simulink model "VehicleFollowing"  (R2020b)
settings: Solver=VariableStepAuto  StartTime=0.0  StopTime=50  RelTol=1e-3
undefined symbols (not defined in the file or in its folder): Discrete, Time
libraries: sim3dautolib x3, vrlib x2, simulink x2, ctrlSharedLib x2, mpcadaslib x2, pid_lib x2, sim3dlib x1, robotmobilelib x1
(part 1 of 2)
settings Model: Creator=Mustafa  LastModifiedBy=JiangHeng
settings SFSimCC: CustomCodeUndefinedFunction=UseInterfaceOnly

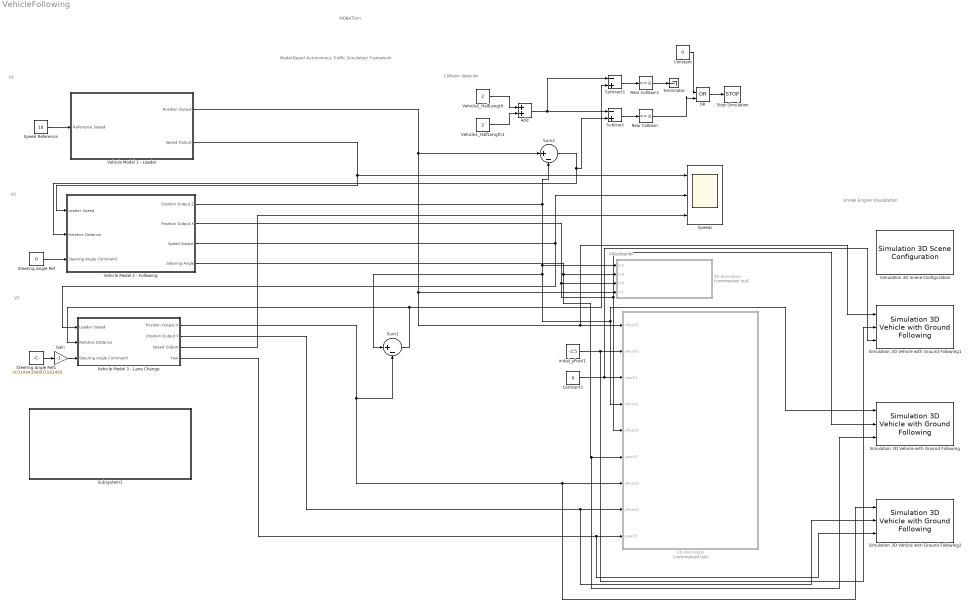
== system VehicleFollowing ==
  note: Unreal Engine Visualization
  note: V1
  note: Visualization
  note: Collision detecion
  note: Model-Based Autonomous Traffic Simulation Framework
  note: MOBATSim
  note: V2
  note: V3
  2D Animation : Subsystem  Commented=on  TreatAsAtomicUnit=on  SystemSampleTime=0.02
  3D Animation : Subsystem  Commented=on
  Add : Sum
  Constant : Constant  Value=0
  Constant1 : Constant  Value=0
  Gain : Gain  Gain=-1
  OR : Logic  Operator=OR  IconShape=distinctive  AllPortsSameDT=off  OutDataTypeStr=boolean
  Rear Collision : simulink/Logic and Bit Operations/Compare To Constant  relop=<=  const=0  OutDataTypeStr=boolean
  Rear Collision1 : simulink/Logic and Bit Operations/Compare To Constant  relop=<=  const=0  OutDataTypeStr=boolean
  Simulation 3D Scene Configuration : sim3dlib/Simulation 3D Scene Configuration  Priority=0  ProjectFormat=Default Scenes  SceneDesc=Straight road  ProjectName=VehicleSimulation.exe  ScenePath=/Game/Maps/HwStrght  vehTagList={'Scene Origin';'SimulinkVehicle1';'SimulinkVehicle2';'SimulinkVehicle3'}  vehTag=SimulinkVehicle3  OpVisEn=off  Ts=0.1  EnableWindow=on  sensorTag=MainCamera1  sensorId=1  sensorName=MainCamera1  mountLoc=Origin  offsetFlag=off  tmountOffset=[0, 0, 0]  rmountOffset=[0, 0, 0]  HorizontalResolution=1280  VerticalResolution=720  HorizontalFOV=60  mountPoint=[0 0 0]  mountOrientation=[0 0 0]  aMode=3  ID=1
      settings: SourceProductBaseCode=DR,UV,VE
  Simulation 3D Vehicle with Ground Following : sim3dautolib/Simulation 3D Vehicle with Ground Following  Priority=-1  PassVehMesh=Small pickup truck  VehColor=Orange  InitialPos=[20, 0, 0]  InitialRot=[0, 0, 0]  ActorName=SimulinkVehicle1  SampleTime=0.1  ActorType=SimulinkVehicle  ID=1  aMode=3  ActorTag=SimulinkVehicle1  CoordinateScheme=ISO  TransformOutportEnabled=off
      settings: SourceProductBaseCode=DR,UV,VE
  Simulation 3D Vehicle with Ground Following1 : sim3dautolib/Simulation 3D Vehicle with Ground Following  Priority=-1  PassVehMesh=Muscle car  VehColor=Red  InitialPos=[40, 0, 0]  InitialRot=[0, 0, 0]  ActorName=SimulinkVehicle2  SampleTime=0.1  ActorType=SimulinkVehicle  ID=2  aMode=3  ActorTag=SimulinkVehicle2  CoordinateScheme=ISO  TransformOutportEnabled=off
      settings: SourceProductBaseCode=DR,UV,VE
  Simulation 3D Vehicle with Ground Following2 : sim3dautolib/Simulation 3D Vehicle with Ground Following  Priority=-1  PassVehMesh=Sedan  VehColor=Silver  InitialPos=[0, 0, 0]  InitialRot=[0, 0, 0]  ActorName=SimulinkVehicle3  SampleTime=0.1  ActorType=SimulinkVehicle  ID=3  aMode=3  ActorTag=SimulinkVehicle3  CoordinateScheme=ISO  TransformOutportEnabled=off
      settings: SourceProductBaseCode=DR,UV,VE
  Speed Reference : Constant  Value=10
  Speeds : Scope  NumInputPorts=3
  Steering Angle Ref : Constant  Value=0
  Steering Angle Ref1 : Constant  Value=-0.01094399007161456
  Stop Simulation : Stop
  Subsystem1 : Subsystem
  Subtract : Sum  Inputs=-+
  Subtract1 : Sum  Inputs=-+
  Sum1 : Sum  Inputs=|+-
  Sum2 : Sum  Inputs=|+-
  Terminator : Terminator
  Vehicle Model 1 - Leader : Subsystem  mask{Pos=40, Speed=20, Disturbance=0}
      mask prompts: Pos "Initial Position"; Speed "Initial Speed"; Disturbance "Leader Vehicle Acceleration Disturbance"
      mask TypeOptions Pos: Initial Position/Value
      mask TypeOptions Speed: Initial Speed/Value
      mask TypeOptions Disturbance: Sine Wave/Amplitude
  Vehicle Model 2 - Following : Subsystem  mask{Pos=20, Speed=25}
      mask prompts: Pos "Initial Position"; Speed "Initial Speed"
      mask TypeOptions Pos: Initial Position Z/Value
      mask TypeOptions Speed: Initial Speed/Value
  Vehicle Model 3 - Lane Change : Subsystem  mask{Pos=0, Speed=10}
      mask prompts: Pos "Initial Position"; Speed "Initial Speed"
      mask TypeOptions Pos: Initial Position X/Value
      mask TypeOptions Speed: Initial Speed/Value
  Vehicle1_HalfLength1 : Constant  Value=2
  Vehicle2_HalfLength : Constant  Value=2
  initial_yPosV1 : Constant  Value=-2.5
  wires:
  Vehicle Model 2 - Following/1(Position Output Z) -> Sum1/1, 2D Animation/4(xPosV2), Simulation 3D Vehicle with Ground Following/1, 3D Animation/1(In2), Sum2/2
  Vehicle Model 2 - Following/3(Speed Output) -> Vehicle Model 3 - Lane Change/1(Leader Speed), Speeds/2
  Speed Reference/1 -> Vehicle Model 1 - Leader/1(Reference Speed)
  Vehicle Model 1 - Leader/1(Position Output) -> Sum2/1, Simulation 3D Vehicle with Ground Following1/1, 2D Animation/1(xPosV1), 3D Animation/4(In1)
  Sum2/1 -> Subtract/2, Vehicle Model 2 - Following/2(Relative Distance)
  Vehicle Model 1 - Leader/2(Speed Output) -> Vehicle Model 2 - Following/1(Leader Speed), Speeds/1
  Steering Angle Ref/1 -> Vehicle Model 2 - Following/3(Steering Angle Command)
  Vehicle Model 2 - Following/2(Position Output X) -> 2D Animation/5(yPosV2), Simulation 3D Vehicle with Ground Following/2, 3D Animation/3(In3)
  Vehicle Model 2 - Following/4(Steering Angle) -> Simulation 3D Vehicle with Ground Following/3, 2D Animation/6(yawV2), 3D Animation/2(In4)
  initial_yPosV1/1 -> Simulation 3D Vehicle with Ground Following1/2, 2D Animation/2(yPosV1)
  Constant1/1 -> Simulation 3D Vehicle with Ground Following1/3, 2D Animation/3(yawV1)
  Vehicle1_HalfLength1/1 -> Add/2
  Vehicle2_HalfLength/1 -> Add/1
  Add/1 -> Subtract1/1, Subtract/1
  Subtract/1 -> Rear Collision/1
  Vehicle Model 3 - Lane Change/1(Position Output X) -> Simulation 3D Vehicle with Ground Following2/1, 2D Animation/7(xPosV3), Sum1/2
  Vehicle Model 3 - Lane Change/2(Position Output Y) -> Simulation 3D Vehicle with Ground Following2/2, 2D Animation/8(yPosV3)
  Vehicle Model 3 - Lane Change/3(Speed Output) -> Speeds/3
  Vehicle Model 3 - Lane Change/4(Yaw) -> Simulation 3D Vehicle with Ground Following2/3, 2D Animation/9(yawV3)
  Sum1/1 -> Vehicle Model 3 - Lane Change/2(Relative Distance), Subtract1/2
  OR/1 -> Stop Simulation/1
  Rear Collision/1 -> OR/2
  Subtract1/1 -> Rear Collision1/1
  Steering Angle Ref1/1 -> Gain/1
  Constant/1 -> OR/1
  Rear Collision1/1 -> Terminator/1
  Gain/1 -> Vehicle Model 3 - Lane Change/3(Steering Angle Command)

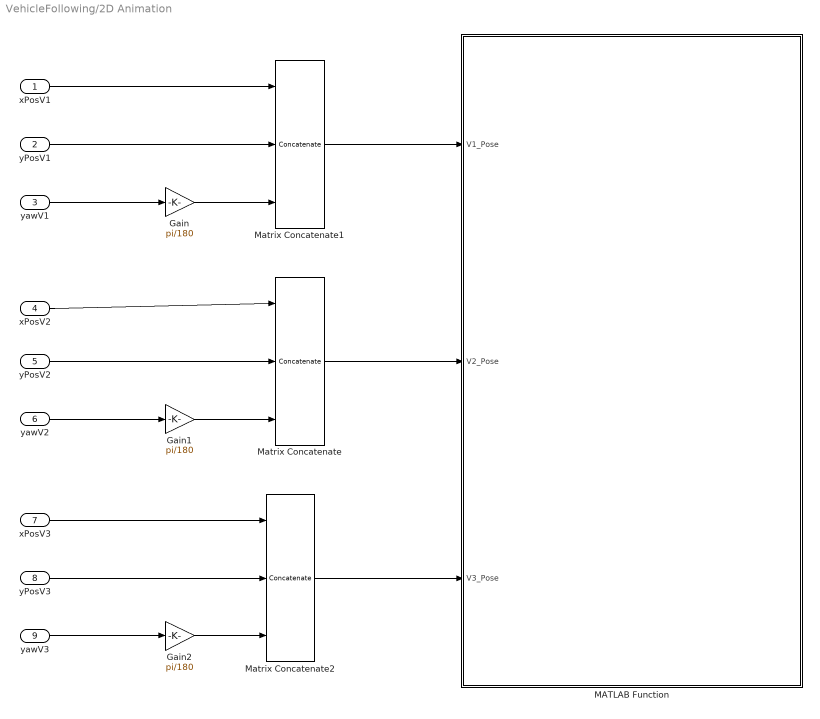
== system VehicleFollowing/2D Animation ==
  xPosV1 : Inport
  yPosV1 : Inport  Port=2
  yawV1 : Inport  Port=3
  xPosV2 : Inport  Port=4
  yPosV2 : Inport  Port=5
  yawV2 : Inport  Port=6
  xPosV3 : Inport  Port=7
  yPosV3 : Inport  Port=8
  yawV3 : Inport  Port=9
  Gain : Gain  Gain=pi/180
  Gain1 : Gain  Gain=pi/180
  Gain2 : Gain  Gain=pi/180
  MATLAB Function : MATLAB Function  TreatAsAtomicUnit=on
      mask init:
      | close all;
      | figure('units','normalized','outerposition',[0 0 1 1]);
      | grid on
      | axis equal
      | hold on
  Matrix Concatenate : Concatenate  NumInputs=3  ConcatenateDimension=2
  Matrix Concatenate1 : Concatenate  NumInputs=3  ConcatenateDimension=2
  Matrix Concatenate2 : Concatenate  NumInputs=3  ConcatenateDimension=2
  wires:
  xPosV2/1 -> Matrix Concatenate/1
  Matrix Concatenate/1 -> MATLAB Function/2(V2_Pose)
  yPosV2/1 -> Matrix Concatenate/2
  yawV2/1 -> Gain1/1
  Matrix Concatenate1/1 -> MATLAB Function/1(V1_Pose)
  xPosV1/1 -> Matrix Concatenate1/1
  yPosV1/1 -> Matrix Concatenate1/2
  yawV1/1 -> Gain/1
  yPosV3/1 -> Matrix Concatenate2/2
  xPosV3/1 -> Matrix Concatenate2/1
  yawV3/1 -> Gain2/1
  Matrix Concatenate2/1 -> MATLAB Function/3(V3_Pose)
  Gain2/1 -> Matrix Concatenate2/3
  Gain1/1 -> Matrix Concatenate/3
  Gain/1 -> Matrix Concatenate1/3

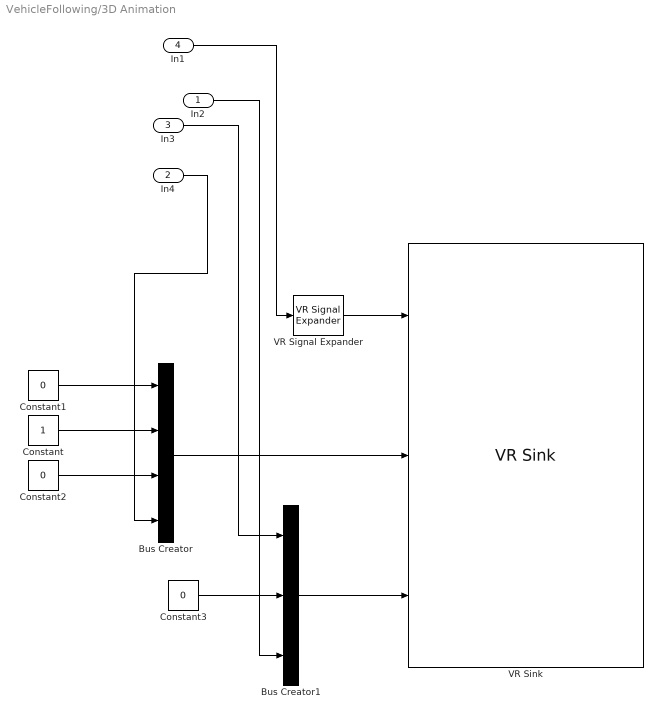
== system VehicleFollowing/3D Animation ==
  In2 : Inport
  In4 : Inport  Port=2
  In3 : Inport  Port=3
  In1 : Inport  Port=4
  Bus Creator : BusCreator  Inputs=4
  Bus Creator1 : BusCreator  Inputs=3
  Constant : Constant
  Constant1 : Constant  Value=0
  Constant2 : Constant  Value=0
  Constant3 : Constant  Value=0
  VR Signal Expander : vrlib/VR Signal Expander  outwidth=3  outidx=[3]
  VR Sink : vrlib/VR Sink  InstantiateOnLoad=on  SampleTime=0.02  ViewEnable=on  RemoteChange=off  RemoteView=off  FieldsWritten=Car_Red.translation.3.1.1.double#Car_Blue.rotation.4.1.1.double#Car_Blue.translation.3.1.1.double  WorldFileName=PlatoonWorld.WRL  AutoView=off  VideoDimensions=[]  AllowVariableSize=off
  wires:
  Constant/1 -> Bus Creator/2
  Constant1/1 -> Bus Creator/1
  Bus Creator1/1 -> VR Sink/3
  In2/1 -> Bus Creator1/3
  Bus Creator/1 -> VR Sink/2
  In4/1 -> Bus Creator/4
  In1/1 -> VR Signal Expander/1
  Constant3/1 -> Bus Creator1/2
  Constant2/1 -> Bus Creator/3
  VR Signal Expander/1 -> VR Sink/1
  In3/1 -> Bus Creator1/1

== system VehicleFollowing/Subsystem1 ==
  Dashboard Scope : DashboardScope
  Gauge : CircularGaugeBlock
  Knob : KnobBlock  ScaleMin=-0.2  ScaleMax=0.2

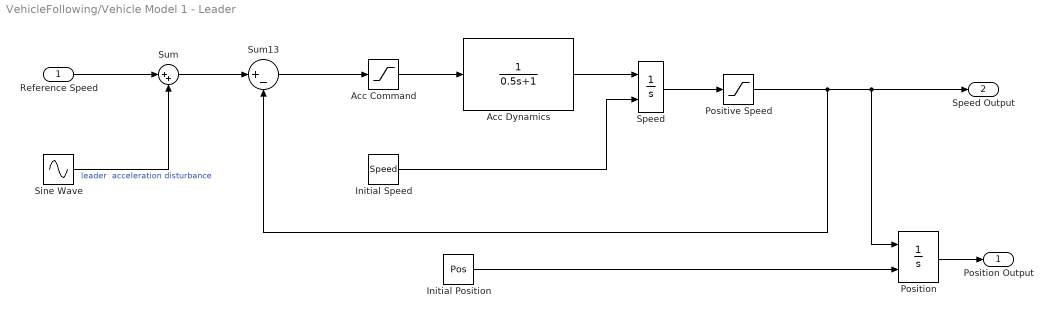
== system VehicleFollowing/Vehicle Model 1 - Leader ==
  Reference Speed : Inport
  Acc Command : Saturate  UpperLimit=2  LowerLimit=-3
  Acc Dynamics : TransferFcn  Denominator=[0.5 1]
  Initial Position : Constant  Value=Pos
  Initial Speed : Constant  Value=Speed
  Position : Integrator  InitialConditionSource=external
  Positive Speed : Saturate  UpperLimit=inf  LowerLimit=0
  Sine Wave : Sin  Amplitude=Disturbance  Frequency=0.2  SampleTime=0.1
  Speed : Integrator  InitialConditionSource=external
  Sum : Sum  Inputs=|++
  Sum13 : Sum  Inputs=|+-
  Position Output : Outport  VectorParamsAs1DForOutWhenUnconnected=off
  Speed Output : Outport  Port=2  VectorParamsAs1DForOutWhenUnconnected=off
  wires:
  Speed/1 -> Positive Speed/1
  Positive Speed/1 -> Sum13/2, Speed Output/1, Position/1
  Initial Position/1 -> Position/2
  Sum13/1 -> Acc Command/1
  Reference Speed/1 -> Sum/1
  Acc Command/1 -> Acc Dynamics/1
  Acc Dynamics/1 -> Speed/1
  Initial Speed/1 -> Speed/2
  Position/1 -> Position Output/1
  Sine Wave/1 -> Sum/2  "leader  acceleration disturbance"
  Sum/1 -> Sum13/1

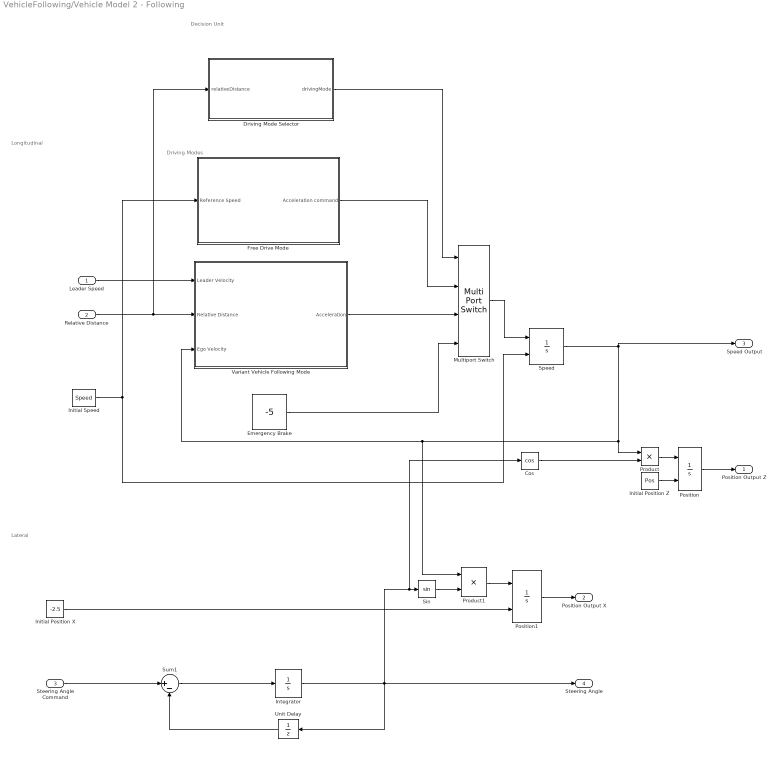
== system VehicleFollowing/Vehicle Model 2 - Following ==
  note: Decision Unit
  note: Driving Modes
  note: Longitudinal
  note: Lateral
  Leader Speed : Inport
  Relative Distance : Inport  Port=2
  Steering Angle Command : Inport  Port=3
  Cos : Trigonometry  Operator=cos
  Driving Mode Selector : Stateflow chart  TreatAsAtomicUnit=on
  Emergency Brake : Constant  Value=-5
  Free Drive Mode : Subsystem
  Initial Position X : Constant  Value=-2.5
  Initial Position Z : Constant  Value=Pos
  Initial Speed : Constant  Value=Speed
  Integrator : Integrator
  Multiport Switch : MultiPortSwitch
  Position : Integrator  InitialConditionSource=external
  Position1 : Integrator  InitialConditionSource=external
  Product : Product
  Product1 : Product
  Sin : Trigonometry
  Speed : Integrator  InitialConditionSource=external  LimitOutput=on  LowerSaturationLimit=0
  Sum1 : Sum  Inputs=|+-
  Unit Delay : UnitDelay  SampleTime=-1  HasFrameUpgradeWarning=on
  Variant Vehicle Following Mode : Subsystem  Variant=on  VariantControlMode=label  LabelModeActiveChoice=MathWorksMPC  mask{ControlType=MathWorksMPC, LabelModeActiveChoice=MathWorksMPC, ControllerBehavior=0.500, Np=10, t_hw=1.4, a_max=2, a_min=-3, fixed_safety_distance=10}
      mask prompts: ControlType "Controller"; LabelModeActiveChoice "Simulink:Variants:LabelComboBox"; ControllerBehavior "Controller Behaviour MathWorks MPC"; Np "Prediction Horizon"; t_hw "Time Headway"; a_max "Maximum Longitudinal Acceleration (m/s^2)"; a_min "Minimum Longitudinal Acceleration (m/s^2)"; fixed_safety_distance "Default Spacing (m)"
      mask TypeOptions ControlType: MathWorksMPC | MPC_quadprog | MPC_quadprog_wKalman | MPC_fmincon | MPC_fmincon_wKalman | PID | CLF_CBF
      mask Callback ControlType:
      | % get the controller name
      | controller = get_param(gcbh,'ControlType');
      | % get the controller behavior from slider
      | maskVariant = Simulink.Mask.get(gcbh);
      | controlBehaviorValue = maskVariant.Parameters(3);
      | predictionHorizonValue = maskVariant.Parameters(4);
      | maximumAccelerationValue = maskVariant.Parameters(6);
      | minimumAccelerationValue = maskVariant.Parameters(7);
      | % if controller is not MathWorks MPC, set controller behavior
      | % slider invisible; if controller is PID, set prediction horizon
      | % and acceleration boundary invisible
      | if strcmp(controller,'MathWorksMPC')
      |     % set the variant according to Popup
      |     set_param(gcbh,'LabelModeActiveChoice','MathWorksMPC');
      |     controlBehaviorValue.set('Visible', 'on');
      |     predictionHorizonValue.set('Visible', 'on');
      |     maximumAccelerationValue.set('Visible', 'on');
      |     minimumAccelerationValue.set('Visible', 'on');
      | elseif strcmp(controller,'MPC_quadprog')
      |     set_param(gcbh,'LabelModeActiveChoice','MPC_quadprog');
      |     controlBehaviorValue.set('Visible', 'off');
      |     predictionHorizonValue.set('Visible', 'on');
      |     maximumAccelerationValue.set('Visible', 'on');
      |     minimumAccelerationValue.set('Visible', 'on');
      | elseif strcmp(controller,'MPC_quadprog_wKalman')
      |     set_param(gcbh,'LabelModeActiveChoice','MPC_quadprog_wKalman');
      |     controlBehaviorValue.set('Visible', 'off');
      |     predictionHorizonValue.set('Visible', 'on');
      |     maximumAccelerationValue.set('Visible', 'on');
      |     minimumAccelerationValue.set('Visible', 'on');
      | elseif strcmp(controller,'MPC_fmincon')
      |     set_param(gcbh,'LabelModeActiveChoice','MPC_fmincon');
      |     controlBehaviorValue.set('Visible', 'off');
      |     predictionHorizonValue.set('Visible', 'on');
      |     maximumAccelerationValue.set('Visible', 'on');
      |     minimumAccelerationValue.set('Visible', 'on');
      | elseif strcmp(controller,'MPC_fmincon_wKalman')
      |     set_param(gcbh,'LabelModeActiveChoice','MPC_fmincon_wKalman');
      |     controlBehaviorValue.set('Visible', 'off');
      |     predictionHorizonValue.set('Visible', 'on');
      |     maximumAccelerationValue.set('Visible', 'on');
      |     minimumAccelerationValue.set('Visible', 'on');
      | elseif strcmp(controller,'PID')
      |     set_param(gcbh,'LabelModeActiveChoice','PID');
      |     controlBehaviorValue.set('Visible', 'off');
      |     predictionHorizonValue.set('Visible', 'off');
      |     maximumAccelerationValue.set('Visible', 'off');
      |     minimumAccelerationValue.set('Visible', 'off');
      | elseif strcmp(controller,'CLF_CBF')
      |     set_param(gcbh,'LabelModeActiveChoice','CLF_CBF');
      |     controlBehaviorValue.set('Visible', 'off');
      |     predictionHorizonValue.set('Visible', 'off');
      |     maximumAccelerationValue.set('Visible', 'on');
      |     minimumAccelerationValue.set('Visible', 'on');
      | end
      mask TypeOptions LabelModeActiveChoice: LabelModeActiveChoice
      mask Callback ControllerBehavior:
      | % set controller behavior of MathWorks MPC according to slider
      | controllerBehavior = get_param(gcbh,'ControllerBehavior');
      | set_param('VehicleFollowing/Vehicle Model 2 - Following/Variant Vehicle Following Mode/MathWorks MPC/Adaptive Cruise Control System', 'ControllerBehavior', controllerBehavior);
      mask TypeOptions Np: MPC fmincon/S-Function/Np | MPC fmincon with Kalman/S-Function/Np | MPC quadprog/S-Function/Np | MPC quadprog with Kalman/S-Function/Np | MathWorks MPC/Adaptive Cruise Control System/PredictionHorizon
      mask TypeOptions t_hw: MPC fmincon/S-Function/t_hw | MPC fmincon with Kalman/S-Function/t_hw | MPC quadprog/S-Function/t_hw | MPC quadprog with Kalman/S-Function/t_hw | MathWorks MPC/Headway Time/Value | PID/Headway Time/Value | CLF//CBF/S-Function/t_hw
      mask TypeOptions a_max: MPC fmincon/S-Function/a_max | MPC fmincon with Kalman/S-Function/a_max | MPC quadprog/S-Function/a_max | MPC quadprog with Kalman/S-Function/a_max | MathWorks MPC/Adaptive Cruise Control System/MaxAcceleration | CLF//CBF/S-Function/a_max
      mask TypeOptions a_min: MPC fmincon/S-Function/a_min | MPC fmincon with Kalman/S-Function/a_min | MPC quadprog/S-Function/a_min | MPC quadprog with Kalman/S-Function/a_min | MathWorks MPC/Adaptive Cruise Control System/MinAcceleration | CLF//CBF/S-Function/a_min
      mask TypeOptions fixed_safety_distance: MPC fmincon/S-Function/fixed_safety_distance | MPC fmincon with Kalman/S-Function/fixed_safety_distance | MPC quadprog/S-Function/fixed_safety_distance | MPC quadprog with Kalman/S-Function/fixed_safety_distance | MathWorks MPC/Adaptive Cruise Control System/DefaultSpacing | PID/Default Spacing/Value | CLF//CBF/S-Function/fixed_safety_distance
      mask DialogControl LabelModeActiveChoice Prompt: Label mode active choice:
  Position Output Z : Outport  VectorParamsAs1DForOutWhenUnconnected=off
  Position Output X : Outport  Port=2  VectorParamsAs1DForOutWhenUnconnected=off
  Speed Output : Outport  Port=3  VectorParamsAs1DForOutWhenUnconnected=off
  Steering Angle : Outport  Port=4  VectorParamsAs1DForOutWhenUnconnected=off
  wires:
  Position/1 -> Position Output Z/1
  Initial Speed/1 -> Free Drive Mode/1(Reference Speed), Speed/2
  Initial Position Z/1 -> Position/2
  Speed/1 -> Speed Output/1, Variant Vehicle Following Mode/3(Ego Velocity), Product1/1, Product/1
  Steering Angle Command/1 -> Sum1/1
  Sum1/1 -> Integrator/1
  Integrator/1 -> Unit Delay/1, Sin/1, Cos/1, Steering Angle/1
  Unit Delay/1 -> Sum1/2
  Initial Position X/1 -> Position1/2
  Cos/1 -> Product/2
  Product/1 -> Position/1
  Sin/1 -> Product1/2
  Product1/1 -> Position1/1
  Position1/1 -> Position Output X/1
  Relative Distance/1 -> Driving Mode Selector/1(relativeDistance), Variant Vehicle Following Mode/2(Relative Distance)
  Leader Speed/1 -> Variant Vehicle Following Mode/1(Leader Velocity)
  Variant Vehicle Following Mode/1(Acceleration) -> Multiport Switch/3
  Multiport Switch/1 -> Speed/1
  Free Drive Mode/1(Acceleration command) -> Multiport Switch/2
  Emergency Brake/1 -> Multiport Switch/4
  Driving Mode Selector/1(drivingMode) -> Multiport Switch/1

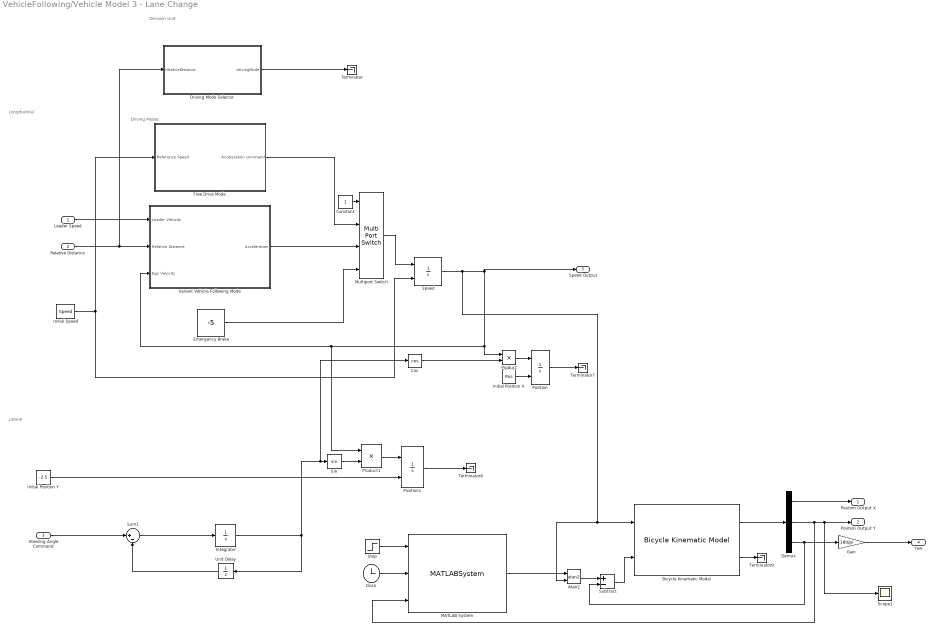
== system VehicleFollowing/Vehicle Model 3 - Lane Change ==
  note: Decision Unit
  note: Driving Modes
  note: Longitudinal
  note: Lateral
  Leader Speed : Inport
  Relative Distance : Inport  Port=2
  Steering Angle Command : Inport  Port=3
  Atan2 : Trigonometry  Operator=atan2
  Bicycle Kinematic Model : robotmobilelib/Bicycle Kinematic Model  VehicleInputs=Vehicle Speed & Steering Angle  WheelBase=3  VehicleSpeedRange=[0 12]  MaxSteeringAngle=pi/4  InitialState=[0; -3; 0]  SimulateUsing=Interpreted execution
      settings: SourceProductBaseCode=RO
  Clock : Clock
  Constant : Constant
  Cos : Trigonometry  Operator=cos
  Demux : Demux  Outputs=3
  Driving Mode Selector : Stateflow chart  TreatAsAtomicUnit=on
  Emergency Brake : Constant  Value=-5
  Free Drive Mode : Subsystem
  Gain : Gain  Gain=180/pi
  Initial Position X : Constant  Value=Pos
  Initial Position Y : Constant  Value=-2.5
  Initial Speed : Constant  Value=Speed
  Integrator : Integrator
  MATLAB System : MATLABSystem  System=LaneChanger  SimulateUsing=Interpreted execution
      mask Type: LaneChanger
      mask Display:
      | disp('LaneChanger');
      | port_label('input',1,'flag');
      | port_label('input',2,'clock');
      | port_label('input',3,'y');
      | port_label('output',1,'latSpeed');
  Multiport Switch : MultiPortSwitch
  Position : Integrator  InitialConditionSource=external
  Position1 : Integrator  InitialConditionSource=external
  Product : Product
  Product1 : Product
  Scope1 : Scope
  Sin : Trigonometry
  Speed : Integrator  InitialConditionSource=external  LimitOutput=on  UpperSaturationLimit=12  LowerSaturationLimit=0
  Step : Step  Time=3  SampleTime=0
  Subtract : Sum  Inputs=+-
  Sum1 : Sum  Inputs=|+-
  Terminator{,7..9} (4 alike) : Terminator
  Unit Delay : UnitDelay  SampleTime=-1  HasFrameUpgradeWarning=on
  Variant Vehicle Following Mode : Subsystem  Variant=on  VariantControlMode=label  LabelModeActiveChoice=PID  mask{ControlType=PID, LabelModeActiveChoice=PID, ControllerBehavior=0.500, Np=10, t_hw=1.4, a_max=2, a_min=-3, fixed_safety_distance=0}
      mask prompts: ControlType "Controller"; LabelModeActiveChoice "Simulink:Variants:LabelComboBox"; ControllerBehavior "Controller Behaviour MathWorks MPC"; Np "Prediction Horizon"; t_hw "Time Headway"; a_max "Maximum Longitudinal Acceleration (m/s^2)"; a_min "Minimum Longitudinal Acceleration (m/s^2)"; fixed_safety_distance "Default Spacing (m)"
      mask TypeOptions ControlType: MathWorksMPC | MPC_quadprog | MPC_quadprog_wKalman | MPC_fmincon | MPC_fmincon_wKalman | PID
      mask Callback ControlType:
      | % get the controller name
      | controller = get_param(gcbh,'ControlType');
      | % get the controller behavior from the slider
      | maskVariant = Simulink.Mask.get(gcbh);
      | controlBehaviorValue = maskVariant.Parameters(3);
      | predictionHorizonValue = maskVariant.Parameters(4);
      | maximumAccelerationValue = maskVariant.Parameters(6);
      | minimumAccelerationValue = maskVariant.Parameters(7);
      | % if controller is not MathWorks MPC, set controller behavior
      | % slider invisible; if controller is PID, set prediction horizon
      | % and acceleration boundary invisible
      | if strcmp(controller,'MathWorksMPC')
      |     % set the variant according to Popup
      |     set_param(gcbh,'LabelModeActiveChoice','MathWorksMPC');
      |     controlBehaviorValue.set('Visible', 'on');
      |     predictionHorizonValue.set('Visible', 'on');
      |     maximumAccelerationValue.set('Visible', 'on');
      |     minimumAccelerationValue.set('Visible', 'on');
      | elseif strcmp(controller,'MPC_quadprog')
      |     set_param(gcbh,'LabelModeActiveChoice','MPC_quadprog');
      |     controlBehaviorValue.set('Visible', 'off');
      |     predictionHorizonValue.set('Visible', 'on');
      |     maximumAccelerationValue.set('Visible', 'on');
      |     minimumAccelerationValue.set('Visible', 'on');
      | elseif strcmp(controller,'MPC_quadprog_wKalman')
      |     set_param(gcbh,'LabelModeActiveChoice','MPC_quadprog_wKalman');
      |     controlBehaviorValue.set('Visible', 'off');
      |     predictionHorizonValue.set('Visible', 'on');
      |     maximumAccelerationValue.set('Visible', 'on');
      |     minimumAccelerationValue.set('Visible', 'on');
      | elseif strcmp(controller,'MPC_fmincon')
      |     set_param(gcbh,'LabelModeActiveChoice','MPC_fmincon');
      |     controlBehaviorValue.set('Visible', 'off');
      |     predictionHorizonValue.set('Visible', 'on');
      |     maximumAccelerationValue.set('Visible', 'on');
      |     minimumAccelerationValue.set('Visible', 'on');
      | elseif strcmp(controller,'MPC_fmincon_wKalman')
      |     set_param(gcbh,'LabelModeActiveChoice','MPC_fmincon_wKalman');
      |     controlBehaviorValue.set('Visible', 'off');
      |     predictionHorizonValue.set('Visible', 'on');
      |     maximumAccelerationValue.set('Visible', 'on');
      |     minimumAccelerationValue.set('Visible', 'on');
      | elseif strcmp(controller,'PID')
      |     set_param(gcbh,'LabelModeActiveChoice','PID');
      |     controlBehaviorValue.set('Visible', 'off');
      |     predictionHorizonValue.set('Visible', 'off');
      |     maximumAccelerationValue.set('Visible', 'off');
      |     minimumAccelerationValue.set('Visible', 'off');
      | end
      mask TypeOptions LabelModeActiveChoice: LabelModeActiveChoice
      mask Callback ControllerBehavior:
      | % set controller behavior of MathWorks MPC according to slider
      | controllerBehavior = get_param(gcbh,'ControllerBehavior');
      | set_param('VehicleFollowing/Vehicle Model 3 - Lane Change/Variant Vehicle Following Mode/MathWorks MPC/Adaptive Cruise Control System', 'ControllerBehavior', controllerBehavior);
      mask TypeOptions Np: MPC fmincon/S-Function/Np | MPC fmincon with Kalman/S-Function/Np | MPC quadprog/S-Function/Np | MPC quadprog with Kalman/S-Function/Np | MathWorks MPC/Adaptive Cruise Control System/PredictionHorizon
      mask TypeOptions t_hw: MPC fmincon/S-Function/t_hw | MPC fmincon with Kalman/S-Function/t_hw | MPC quadprog/S-Function/t_hw | MPC quadprog with Kalman/S-Function/t_hw | MathWorks MPC/Headway Time/Value | PID/Headway Time/Value
      mask TypeOptions a_max: MPC fmincon/S-Function/a_max | MPC fmincon with Kalman/S-Function/a_max | MPC quadprog/S-Function/a_max | MPC quadprog with Kalman/S-Function/a_max | MathWorks MPC/Adaptive Cruise Control System/MaxAcceleration
      mask TypeOptions a_min: MPC fmincon/S-Function/a_min | MPC fmincon with Kalman/S-Function/a_min | MPC quadprog/S-Function/a_min | MPC quadprog with Kalman/S-Function/a_min | MathWorks MPC/Adaptive Cruise Control System/MinAcceleration
      mask TypeOptions fixed_safety_distance: MPC fmincon/S-Function/fixed_safety_distance | MPC fmincon with Kalman/S-Function/fixed_safety_distance | MPC quadprog/S-Function/fixed_safety_distance | MPC quadprog with Kalman/S-Function/fixed_safety_distance | MathWorks MPC/Adaptive Cruise Control System/DefaultSpacing | PID/Default Spacing/Value
      mask DialogControl LabelModeActiveChoice Prompt: Label mode active choice:
  Position Output X : Outport  VectorParamsAs1DForOutWhenUnconnected=off
  Position Output Y : Outport  Port=2  VectorParamsAs1DForOutWhenUnconnected=off
  Speed Output : Outport  Port=3  VectorParamsAs1DForOutWhenUnconnected=off
  Yaw : Outport  Port=4  VectorParamsAs1DForOutWhenUnconnected=off
  wires:
  Initial Speed/1 -> Free Drive Mode/1(Reference Speed), Speed/2
  Initial Position X/1 -> Position/2
  Speed/1 -> Atan2/2, Bicycle Kinematic Model/1, Speed Output/1, Variant Vehicle Following Mode/3(Ego Velocity), Product1/1, Product/1
  Sum1/1 -> Integrator/1
  Integrator/1 -> Unit Delay/1, Sin/1, Cos/1
  Unit Delay/1 -> Sum1/2
  Initial Position Y/1 -> Position1/2
  Cos/1 -> Product/2
  Product/1 -> Position/1
  Sin/1 -> Product1/2
  Product1/1 -> Position1/1
  Relative Distance/1 -> Driving Mode Selector/1(relativeDistance), Variant Vehicle Following Mode/2(Relative Distance)
  Leader Speed/1 -> Variant Vehicle Following Mode/1(Leader Velocity)
  Variant Vehicle Following Mode/1(Acceleration) -> Multiport Switch/3
  Multiport Switch/1 -> Speed/1
  Free Drive Mode/1(Acceleration command) -> Multiport Switch/2
  Emergency Brake/1 -> Multiport Switch/4
  Driving Mode Selector/1(drivingMode) -> Terminator/1
  Constant/1 -> Multiport Switch/1
  Position/1 -> Terminator7/1
  Position1/1 -> Terminator8/1
  Gain/1 -> Yaw/1
  Bicycle Kinematic Model/1 -> Demux/1
  Bicycle Kinematic Model/2 -> Terminator9/1
  Demux/3 -> Subtract/2, Gain/1
  Demux/2 -> MATLAB System/3, Scope1/1, Position Output Y/1
  Demux/1 -> Position Output X/1
  Steering Angle Command/1 -> Sum1/1
  Step/1 -> MATLAB System/1
  Clock/1 -> MATLAB System/2
  MATLAB System/1 -> Atan2/1
  Atan2/1 -> Subtract/1
  Subtract/1 -> Bicycle Kinematic Model/2

== system VehicleFollowing/Vehicle Model 2 - Following/Free Drive Mode ==
  Reference Speed : Inport
  Acc Command : Saturate  UpperLimit=2  LowerLimit=-3
  Acc Dynamics : TransferFcn  Denominator=[0.5 1]
  Sum13 : Sum  Inputs=|+-
  Acceleration command : Outport
  wires:
  Sum13/1 -> Acc Command/1
  Acc Dynamics/1 -> Acceleration command/1, Sum13/2
  Reference Speed/1 -> Sum13/1
  Acc Command/1 -> Acc Dynamics/1

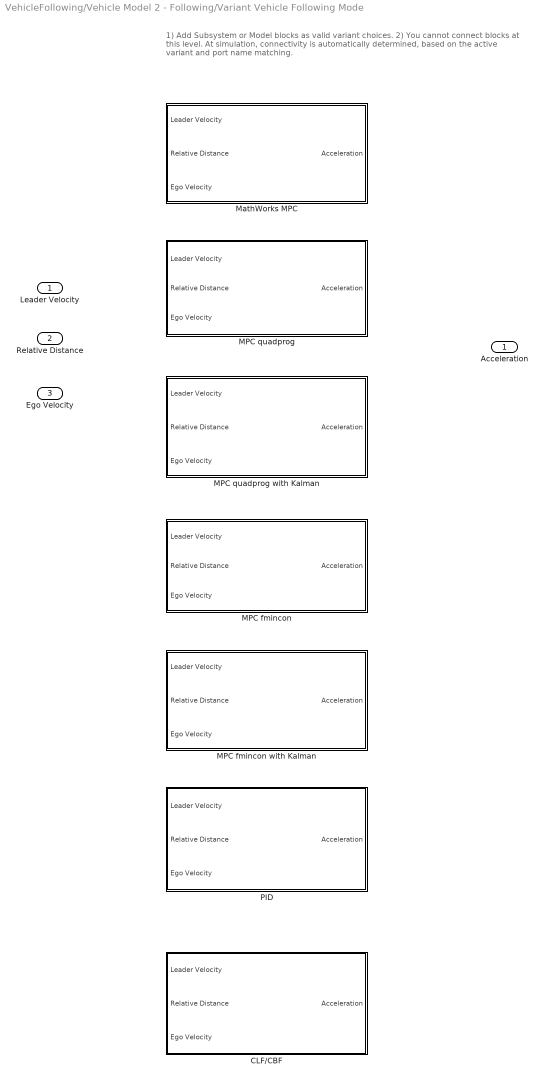
== system VehicleFollowing/Vehicle Model 2 - Following/Variant Vehicle Following Mode ==
  note: 1) Add Subsystem or Model blocks as valid variant choices.
      | 2) You cannot connect blocks at this level. At simulation, connectivity is automatically
      | determined, based on the active variant and port name matching.
  Leader Velocity : Inport
  Relative Distance : Inport  Port=2
  Ego Velocity : Inport  Port=3
  CLF/CBF : Subsystem  VariantControl=CLF_CBF
  MPC fmincon : Subsystem  VariantControl=MPC_fmincon
  MPC fmincon with Kalman : Subsystem  VariantControl=MPC_fmincon_wKalman
  MPC quadprog : Subsystem  VariantControl=MPC_quadprog
  MPC quadprog with Kalman : Subsystem  VariantControl=MPC_quadprog_wKalman
  MathWorks MPC : Subsystem  VariantControl=MathWorksMPC
  PID : Subsystem  VariantControl=PID
  Acceleration : Outport

== system VehicleFollowing/Vehicle Model 3 - Lane Change/Free Drive Mode ==
  Reference Speed : Inport
  Acc Command : Saturate  UpperLimit=2  LowerLimit=-3
  Acc Dynamics : TransferFcn  Denominator=[0.5 1]
  Sum13 : Sum  Inputs=|+-
  Acceleration command : Outport
  wires:
  Sum13/1 -> Acc Command/1
  Acc Dynamics/1 -> Acceleration command/1, Sum13/2
  Reference Speed/1 -> Sum13/1
  Acc Command/1 -> Acc Dynamics/1

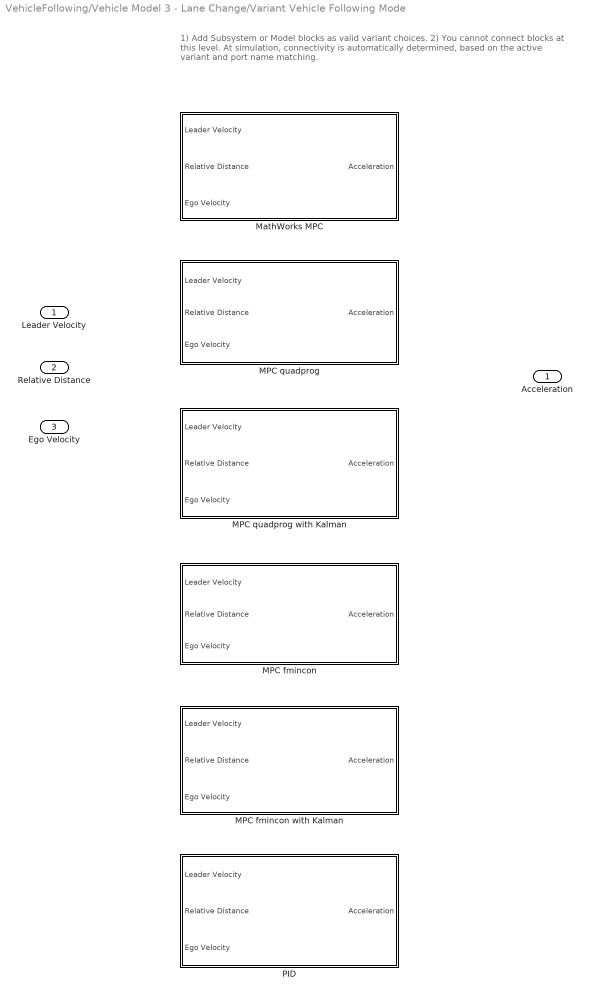
== system VehicleFollowing/Vehicle Model 3 - Lane Change/Variant Vehicle Following Mode ==
  note: 1) Add Subsystem or Model blocks as valid variant choices.
      | 2) You cannot connect blocks at this level. At simulation, connectivity is automatically
      | determined, based on the active variant and port name matching.
  Leader Velocity : Inport
  Relative Distance : Inport  Port=2
  Ego Velocity : Inport  Port=3
  MPC fmincon : Subsystem  VariantControl=MPC_fmincon
  MPC fmincon with Kalman : Subsystem  VariantControl=MPC_fmincon_wKalman
  MPC quadprog : Subsystem  VariantControl=MPC_quadprog
  MPC quadprog with Kalman : Subsystem  VariantControl=MPC_quadprog_wKalman
  MathWorks MPC : Subsystem  VariantControl=MathWorksMPC
  PID : Subsystem  VariantControl=PID
  Acceleration : Outport

== system VehicleFollowing/Vehicle Model 2 - Following/Variant Vehicle Following Mode/CLF//CBF ==
  Leader Velocity : Inport
  Relative Distance : Inport  Port=2
  Ego Velocity : Inport  Port=3
  Mux : Mux  Inputs=3
  S-Function : S-Function  FunctionName=CLFCBF  Parameters=t_hw, a_max, a_min, fixed_safety_distance  SFunctionDeploymentMode=off  EnableBusSupport=off  mask{t_hw=t_hw, a_max=a_max, a_min=a_min, fixed_safety_distance=fixed_safety_distance}
      mask prompts: t_hw "Time Headway (s)"; a_max "Maximum Longitudinal Acceleration (m/s^2)"; a_min "Minimum Longitudinal Acceleration (m/s^2)"; fixed_safety_distance "Default Spacing (m)"
  Sum13 : Sum  Inputs=|+-
  Acceleration : Outport
  wires:
  Mux/1 -> S-Function/1
  Leader Velocity/1 -> Sum13/1
  Ego Velocity/1 -> Sum13/2, Mux/3
  Relative Distance/1 -> Mux/1  "relative distance my MPC"
  Sum13/1 -> Mux/2
  S-Function/1 -> Acceleration/1

== system VehicleFollowing/Vehicle Model 2 - Following/Variant Vehicle Following Mode/MPC fmincon ==
  Leader Velocity : Inport
  Relative Distance : Inport  Port=2
  Ego Velocity : Inport  Port=3
  Mux : Mux  Inputs=3
  S-Function : S-Function  FunctionName=MPC_fmincon  Parameters=Np, t_hw, a_max, a_min, fixed_safety_distance  SFunctionDeploymentMode=off  EnableBusSupport=off  mask{Np=Np, t_hw=t_hw, a_max=a_max, a_min=a_min, fixed_safety_distance=fixed_safety_distance}
      mask prompts: Np "Prediction Horizon (s)"; t_hw "Time Headway"; a_max "Maximum Longitudinal Acceleration (m/s^2)"; a_min "Minimum Longitudinal Acceleration (m/s^2)"; fixed_safety_distance "Default Spacing (m)"
  Sum13 : Sum  Inputs=|+-
  Acceleration : Outport
  wires:
  Sum13/1 -> Mux/2
  Ego Velocity/1 -> Sum13/2, Mux/3
  Leader Velocity/1 -> Sum13/1
  Mux/1 -> S-Function/1
  Relative Distance/1 -> Mux/1  "relative distance my MPC"
  S-Function/1 -> Acceleration/1

== system VehicleFollowing/Vehicle Model 2 - Following/Variant Vehicle Following Mode/MPC fmincon with Kalman ==
  Leader Velocity : Inport
  Relative Distance : Inport  Port=2
  Ego Velocity : Inport  Port=3
  Kalman Filter : ctrlSharedLib/Kalman Filter  TimeDomain=Discrete-Time  UseCurrentEstimator=on  ModelSource=Individual A, B, C, D matrices  ModelSourceVariable=ss(0.95,1,1,0,1)  A=|  B=[-0.5^3; -0.5; 0.5];  C="[1 0 0; 0 1  0; 0 0 1];"  D=0  NumberOfStates=1  NumberOfInputs=1  NumberOfOutputs=1  InitialEstimateSource=Dialog  X0=[0;0;0]  P0=10  UseK=off  UseGH=on  NumberOfProcessNoiseInputs=1  G=[1 0 0;0 1 0;0 0 1]  TimeInvariantG=on  H=[1 0 0;0 1 0; 0 0 1]  TimeInvariantH=on  Q="[0.01   0    0;0 0.01  0;0   0   0.01];"  TimeInvariantQ=on  R=|  TimeInvariantR=on  N=0  TimeInvariantN=on  AddInputPort=on  AddEnablePort=off  OutputEstimatedY=off  OutputP=off  Ts=0.5
      A=|
      | [1 0.5 0; 0 1  0;
      |  0 0  1];
      R=|
      | [0.1  0  0;
      |  0  0.1  0;     0  0  0.1];
  Mux : Mux  Inputs=3
  Rate Transition : RateTransition  OutPortSampleTime=0.5
  S-Function : S-Function  FunctionName=MPC_fmincon_wKalman  Parameters=Np, t_hw, a_max, a_min, fixed_safety_distance  SFunctionDeploymentMode=off  EnableBusSupport=off  mask{Np=Np, t_hw=t_hw, a_max=a_max, a_min=a_min, fixed_safety_distance=fixed_safety_distance}
      mask prompts: Np "Prediction Horizon"; t_hw "Time Headway (s)"; a_max "Maximum Longitudinal Acceleration (m/s^2)"; a_min "Minimum Longitudinal Acceleration (m/s^2)"; fixed_safety_distance "Default Spacing (m)"
  Sum13 : Sum  Inputs=|+-
  Acceleration : Outport
  wires:
  Sum13/1 -> Mux/2
  Ego Velocity/1 -> Sum13/2, Mux/3
  Leader Velocity/1 -> Sum13/1
  Mux/1 -> Rate Transition/1
  Relative Distance/1 -> Mux/1  "relative distance my MPC"
  S-Function/1 -> Kalman Filter/1, Acceleration/1
  Rate Transition/1 -> Kalman Filter/2
  Kalman Filter/1 -> S-Function/1

== system VehicleFollowing/Vehicle Model 2 - Following/Variant Vehicle Following Mode/MPC quadprog ==
  Leader Velocity : Inport
  Relative Distance : Inport  Port=2
  Ego Velocity : Inport  Port=3
  Mux : Mux  Inputs=3
  S-Function : S-Function  FunctionName=MPC_quadprog  Parameters=Np, t_hw, a_max, a_min, fixed_safety_distance  SFunctionDeploymentMode=off  EnableBusSupport=off  mask{Np=Np, t_hw=t_hw, a_max=a_max, a_min=a_min, fixed_safety_distance=fixed_safety_distance}
      mask prompts: Np "Prediction Horizon"; t_hw "Time Headway (s)"; a_max "Maximum Longitudinal Acceleration (m/s^2)"; a_min "Minimum Longitudinal Acceleration (m/s^2)"; fixed_safety_distance "Default Spacing (m)"
  Sum13 : Sum  Inputs=|+-
  Acceleration : Outport
  wires:
  Relative Distance/1 -> Mux/1  "relative distance my MPC"
  Ego Velocity/1 -> Sum13/2, Mux/3
  Sum13/1 -> Mux/2
  Mux/1 -> S-Function/1
  Leader Velocity/1 -> Sum13/1
  S-Function/1 -> Acceleration/1

== system VehicleFollowing/Vehicle Model 2 - Following/Variant Vehicle Following Mode/MPC quadprog with Kalman ==
  Leader Velocity : Inport
  Relative Distance : Inport  Port=2
  Ego Velocity : Inport  Port=3
  Kalman Filter : ctrlSharedLib/Kalman Filter  TimeDomain=Discrete-Time  UseCurrentEstimator=on  ModelSource=Individual A, B, C, D matrices  ModelSourceVariable=ss(0.95,1,1,0,1)  A=|  B=[-0.5^3; -0.5; 0.5];  C="[1 0 0; 0 1  0; 0 0 1];"  D=0  NumberOfStates=1  NumberOfInputs=1  NumberOfOutputs=1  InitialEstimateSource=Dialog  X0=[0;0;0]  P0=10  UseK=off  UseGH=on  NumberOfProcessNoiseInputs=1  G=[1 0 0;0 1 0;0 0 1]  TimeInvariantG=on  H=[1 0 0;0 1 0; 0 0 1]  TimeInvariantH=on  Q="[0.01   0    0;0 0.01  0;0   0   0.01];"  TimeInvariantQ=on  R=|  TimeInvariantR=on  N=0  TimeInvariantN=on  AddInputPort=on  AddEnablePort=off  OutputEstimatedY=off  OutputP=off  Ts=0.5
      A=|
      | [1 0.5 0; 0 1  0;
      |  0 0  1];
      R=|
      | [0.1  0  0;
      |  0  0.1  0;     0  0  0.1];
  Mux : Mux  Inputs=3
  Rate Transition : RateTransition  OutPortSampleTime=0.5
  S-Function : S-Function  FunctionName=MPC_quadprog_wKalman  Parameters=Np, t_hw, a_max, a_min, fixed_safety_distance  SFunctionDeploymentMode=off  EnableBusSupport=off  mask{Np=Np, t_hw=t_hw, a_max=a_max, a_min=a_min, fixed_safety_distance=fixed_safety_distance}
      mask prompts: Np "Prediction Horizon"; t_hw "Time Headway (s)"; a_max "Maximum Longitudinal Acceleration (m/s^2)"; a_min "Minimum Longitudinal Acceleration (m/s^2)"; fixed_safety_distance "Default Spacing (m)"
  Sum13 : Sum  Inputs=|+-
  Acceleration : Outport
  wires:
  Sum13/1 -> Mux/2
  Ego Velocity/1 -> Sum13/2, Mux/3
  Leader Velocity/1 -> Sum13/1
  Mux/1 -> Rate Transition/1
  Relative Distance/1 -> Mux/1  "relative distance my MPC"
  S-Function/1 -> Kalman Filter/1, Acceleration/1
  Rate Transition/1 -> Kalman Filter/2
  Kalman Filter/1 -> S-Function/1

== system VehicleFollowing/Vehicle Model 2 - Following/Variant Vehicle Following Mode/MathWorks MPC ==
  Leader Velocity : Inport
  Relative Distance : Inport  Port=2
  Ego Velocity : Inport  Port=3
  Adaptive Cruise Control System : mpcadaslib/Adaptive Cruise Control System  EgoModel=tf(1,[1,0])  InitialEgoVelocity=10  DefaultSpacing=fixed_safety_distance  MaxVelocity=30  MinAcceleration=a_min  amin_ext=off  MaxAcceleration=a_max  amax_ext=off  Ts=0.5  PredictionHorizon=Np  ControllerBehavior=0.500  suboptimal=off  maxiter=100  datatypeopt=double  optmode=off  trackmode=off
  Headway Time : Constant  Value=t_hw
  Reference Velocity : Constant  Value=30
  Sum13 : Sum  Inputs=+-|
  Acceleration : Outport
  wires:
  Reference Velocity/1 -> Adaptive Cruise Control System/1
  Headway Time/1 -> Adaptive Cruise Control System/2
  Relative Distance/1 -> Adaptive Cruise Control System/4  "relative distance MathWorks"
  Leader Velocity/1 -> Sum13/1
  Sum13/1 -> Adaptive Cruise Control System/5
  Ego Velocity/1 -> Adaptive Cruise Control System/3, Sum13/2
  Adaptive Cruise Control System/1 -> Acceleration/1  "MathWork"

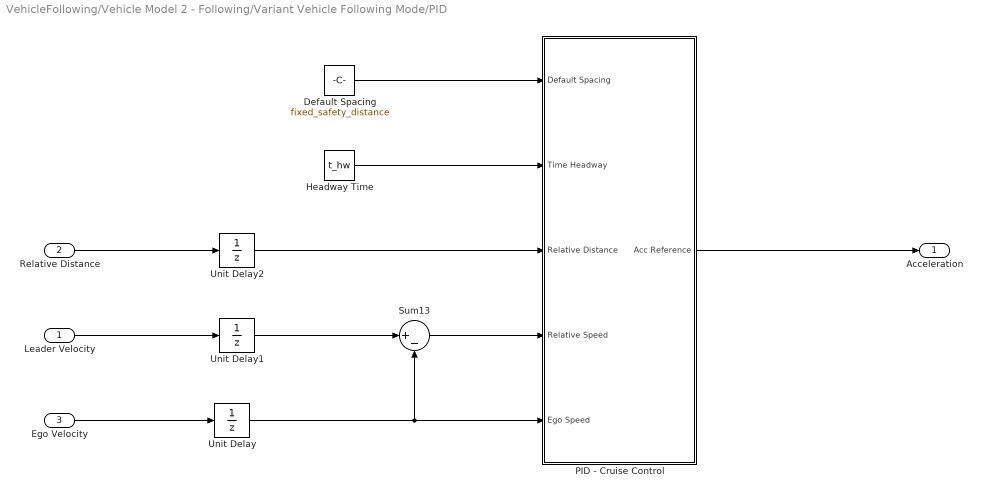
== system VehicleFollowing/Vehicle Model 2 - Following/Variant Vehicle Following Mode/PID ==
  Leader Velocity : Inport
  Relative Distance : Inport  Port=2
  Ego Velocity : Inport  Port=3
  Default Spacing : Constant  Value=fixed_safety_distance
  Headway Time : Constant  Value=t_hw
  PID - Cruise Control : Subsystem
  Sum13 : Sum  Inputs=|+-
  Unit Delay : UnitDelay  SampleTime=-1  HasFrameUpgradeWarning=on
  Unit Delay1 : UnitDelay  SampleTime=-1  HasFrameUpgradeWarning=on
  Unit Delay2 : UnitDelay  SampleTime=-1  HasFrameUpgradeWarning=on
  Acceleration : Outport
  wires:
  Unit Delay2/1 -> PID - Cruise Control/3(Relative Distance)
  Relative Distance/1 -> Unit Delay2/1
  PID - Cruise Control/1(Acc Reference) -> Acceleration/1
  Ego Velocity/1 -> Unit Delay/1
  Unit Delay/1 -> Sum13/2, PID - Cruise Control/5(Ego Speed)
  Unit Delay1/1 -> Sum13/1
  Default Spacing/1 -> PID - Cruise Control/1(Default Spacing)
  Sum13/1 -> PID - Cruise Control/4(Relative Speed)
  Headway Time/1 -> PID - Cruise Control/2(Time Headway)
  Leader Velocity/1 -> Unit Delay1/1

== system VehicleFollowing/Vehicle Model 3 - Lane Change/Variant Vehicle Following Mode/MPC fmincon ==
  Leader Velocity : Inport
  Relative Distance : Inport  Port=2
  Ego Velocity : Inport  Port=3
  Mux : Mux  Inputs=3
  S-Function : S-Function  FunctionName=MPC_fmincon  Parameters=Np, t_hw, a_max, a_min, fixed_safety_distance  SFunctionDeploymentMode=off  EnableBusSupport=off  mask{Np=Np, t_hw=t_hw, a_max=a_max, a_min=a_min, fixed_safety_distance=fixed_safety_distance}
      mask prompts: Np "Prediction Horizon"; t_hw "Time Headway (s)"; a_max "Maximum Longitudinal Acceleration (m/s^2)"; a_min "Minimum Longitudinal Acceleration (m/s^2)"; fixed_safety_distance "Default Spacing (m)"
  Sum13 : Sum  Inputs=|+-
  Acceleration : Outport
  wires:
  Sum13/1 -> Mux/2
  Ego Velocity/1 -> Sum13/2, Mux/3
  Leader Velocity/1 -> Sum13/1
  Mux/1 -> S-Function/1
  Relative Distance/1 -> Mux/1  "relative distance my MPC"
  S-Function/1 -> Acceleration/1

== system VehicleFollowing/Vehicle Model 3 - Lane Change/Variant Vehicle Following Mode/MPC fmincon with Kalman ==
  Leader Velocity : Inport
  Relative Distance : Inport  Port=2
  Ego Velocity : Inport  Port=3
  Mux : Mux  Inputs=3
  S-Function : S-Function  FunctionName=MPC_fmincon_wKalman  Parameters=Np, t_hw, a_max, a_min, fixed_safety_distance  SFunctionDeploymentMode=off  EnableBusSupport=off  mask{Np=Np, t_hw=t_hw, a_max=a_max, a_min=a_min, fixed_safety_distance=fixed_safety_distance}
      mask prompts: Np "Prediction Horizon"; t_hw "Time Headway (s)"; a_max "Maximum Longitudinal Acceleration (m/s^2)"; a_min "Minimum Longitudinal Acceleration (m/s^2)"; fixed_safety_distance "Default Spacing (m)"
  Sum13 : Sum  Inputs=|+-
  Acceleration : Outport
  wires:
  Sum13/1 -> Mux/2
  Ego Velocity/1 -> Sum13/2, Mux/3
  Leader Velocity/1 -> Sum13/1
  Mux/1 -> S-Function/1
  Relative Distance/1 -> Mux/1  "relative distance my MPC"
  S-Function/1 -> Acceleration/1

== system VehicleFollowing/Vehicle Model 3 - Lane Change/Variant Vehicle Following Mode/MPC quadprog ==
  Leader Velocity : Inport
  Relative Distance : Inport  Port=2
  Ego Velocity : Inport  Port=3
  Mux : Mux  Inputs=3
  S-Function : S-Function  FunctionName=MPC_quadprog  Parameters=Np, t_hw, a_max, a_min, fixed_safety_distance  SFunctionDeploymentMode=off  EnableBusSupport=off  mask{Np=Np, t_hw=t_hw, a_max=a_max, a_min=a_min, fixed_safety_distance=fixed_safety_distance}
      mask prompts: Np "Prediction Horizon"; t_hw "Time Headway (m)"; a_max "Maximum Longitudinal Acceleration (m/s^2)"; a_min "Minimum Longitudinal Acceleration (m/s^2)"; fixed_safety_distance "Default Spacing (m)"
  Sum13 : Sum  Inputs=|+-
  Acceleration : Outport
  wires:
  Relative Distance/1 -> Mux/1  "relative distance my MPC"
  Ego Velocity/1 -> Sum13/2, Mux/3
  Sum13/1 -> Mux/2
  Mux/1 -> S-Function/1
  Leader Velocity/1 -> Sum13/1
  S-Function/1 -> Acceleration/1

== system VehicleFollowing/Vehicle Model 3 - Lane Change/Variant Vehicle Following Mode/MPC quadprog with Kalman ==
  Leader Velocity : Inport
  Relative Distance : Inport  Port=2
  Ego Velocity : Inport  Port=3
  Mux : Mux  Inputs=3
  S-Function : S-Function  FunctionName=MPC_quadprog_wKalman  Parameters=Np, t_hw, a_max, a_min, fixed_safety_distance  SFunctionDeploymentMode=off  EnableBusSupport=off  mask{Np=Np, t_hw=t_hw, a_max=a_max, a_min=a_min, fixed_safety_distance=fixed_safety_distance}
      mask prompts: Np "Prediction Horizon"; t_hw "Time Headway (s)"; a_max "Maximum Longitudinal Acceleration (m/s^2)"; a_min "Minimum Longitudinal Acceleration (m/s^2)"; fixed_safety_distance "Default Spacing (m)"
  Sum13 : Sum  Inputs=|+-
  Acceleration : Outport
  wires:
  Sum13/1 -> Mux/2
  Ego Velocity/1 -> Sum13/2, Mux/3
  Leader Velocity/1 -> Sum13/1
  Mux/1 -> S-Function/1
  Relative Distance/1 -> Mux/1  "relative distance my MPC"
  S-Function/1 -> Acceleration/1

== system VehicleFollowing/Vehicle Model 3 - Lane Change/Variant Vehicle Following Mode/MathWorks MPC ==
  Leader Velocity : Inport
  Relative Distance : Inport  Port=2
  Ego Velocity : Inport  Port=3
  Adaptive Cruise Control System : mpcadaslib/Adaptive Cruise Control System  EgoModel=tf(1,[1,0])  InitialEgoVelocity=10  DefaultSpacing=fixed_safety_distance  MaxVelocity=30  MinAcceleration=a_min  amin_ext=off  MaxAcceleration=a_max  amax_ext=off  Ts=0.5  PredictionHorizon=Np  ControllerBehavior=0.500  suboptimal=off  maxiter=100  datatypeopt=double  optmode=off  trackmode=off
  Headway Time : Constant  Value=t_hw
  Reference Velocity : Constant  Value=30
  Sum13 : Sum  Inputs=+-|
  Acceleration : Outport
  wires:
  Reference Velocity/1 -> Adaptive Cruise Control System/1
  Headway Time/1 -> Adaptive Cruise Control System/2
  Relative Distance/1 -> Adaptive Cruise Control System/4  "relative distance MathWorks"
  Leader Velocity/1 -> Sum13/1
  Sum13/1 -> Adaptive Cruise Control System/5
  Ego Velocity/1 -> Adaptive Cruise Control System/3, Sum13/2
  Adaptive Cruise Control System/1 -> Acceleration/1  "MathWork"

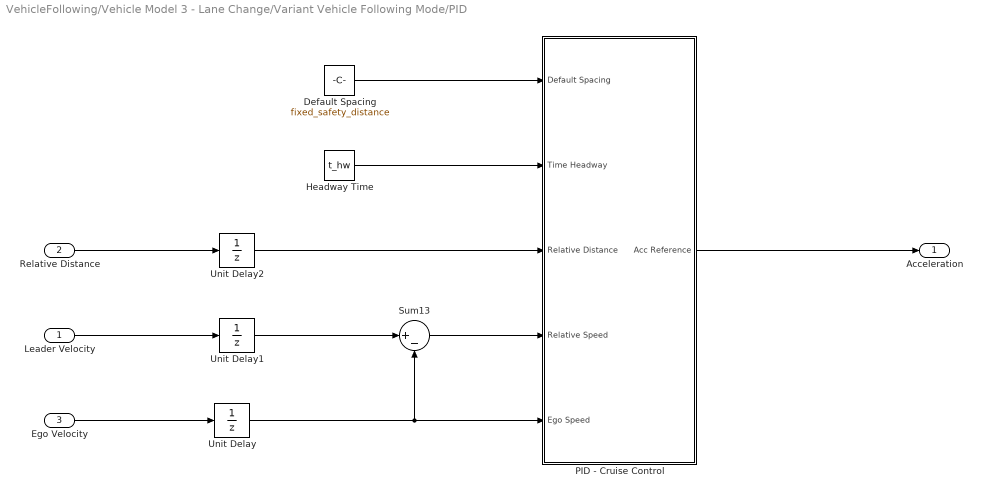
== system VehicleFollowing/Vehicle Model 3 - Lane Change/Variant Vehicle Following Mode/PID ==
  Leader Velocity : Inport
  Relative Distance : Inport  Port=2
  Ego Velocity : Inport  Port=3
  Default Spacing : Constant  Value=fixed_safety_distance
  Headway Time : Constant  Value=t_hw
  PID - Cruise Control : Subsystem
  Sum13 : Sum  Inputs=|+-
  Unit Delay : UnitDelay  SampleTime=-1  HasFrameUpgradeWarning=on
  Unit Delay1 : UnitDelay  SampleTime=-1  HasFrameUpgradeWarning=on
  Unit Delay2 : UnitDelay  SampleTime=-1  HasFrameUpgradeWarning=on
  Acceleration : Outport
  wires:
  Unit Delay2/1 -> PID - Cruise Control/3(Relative Distance)
  Relative Distance/1 -> Unit Delay2/1
  PID - Cruise Control/1(Acc Reference) -> Acceleration/1
  Ego Velocity/1 -> Unit Delay/1
  Unit Delay/1 -> Sum13/2, PID - Cruise Control/5(Ego Speed)
  Unit Delay1/1 -> Sum13/1
  Default Spacing/1 -> PID - Cruise Control/1(Default Spacing)
  Sum13/1 -> PID - Cruise Control/4(Relative Speed)
  Headway Time/1 -> PID - Cruise Control/2(Time Headway)
  Leader Velocity/1 -> Unit Delay1/1

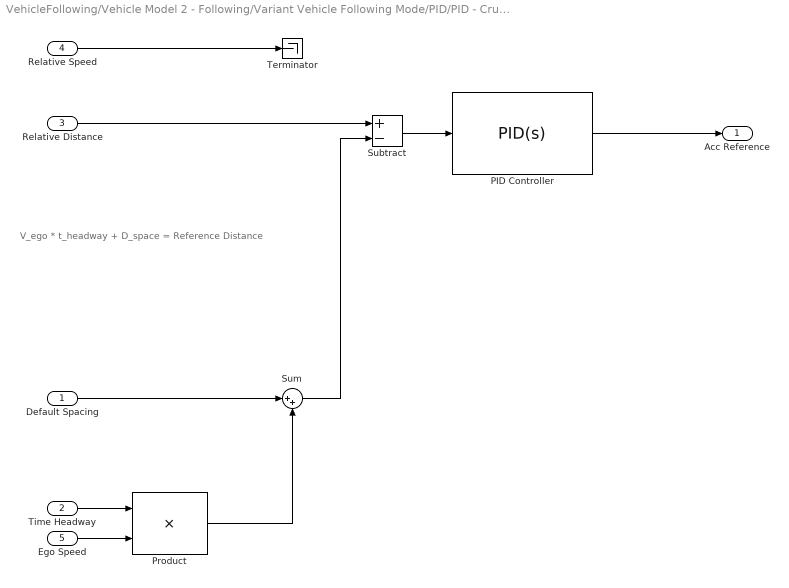
== system VehicleFollowing/Vehicle Model 2 - Following/Variant Vehicle Following Mode/PID/PID - Cruise Control ==
  note: V_ego * t_headway + D_space = Reference Distance
  Default Spacing : Inport
  Time Headway : Inport  Port=2
  Relative Distance : Inport  Port=3
  Relative Speed : Inport  Port=4
  Ego Speed : Inport  Port=5
  PID Controller : pid_lib/PID Controller  Controller=PID  Form=Parallel  TimeDomain=Continuous-time  UseExternalTs=off  SampleTime=-1  IntegratorMethod=Forward Euler  FilterMethod=Forward Euler  ControllerParametersSource=internal  P=2  I=0.04  D=2.1  UseFilter=on  N=230  TunerSelectOption=Transfer Function Based (PID Tuner App)  InitialConditionSource=internal  InitialConditionForIntegrator=0  InitialConditionForFilter=0  DifferentiatorICPrevScaledInput=0  ExternalReset=none  TrackingMode=off  Kt=1  LimitOutput=on  SatLimitsSource=internal  UpperSaturationLimit=2  LowerSaturationLimit=-3  LinearizeAsGain=on  AntiWindupMode=clamping  Kb=1  POutMin=[]  POutMax=[]  IOutMin=[]  IOutMax=[]  DOutMin=[]  DOutMax=[]  NOutMin=[]  NOutMax=[]  SumOutMin=[]  SumOutMax=[]  SaturationOutMin=[]  SaturationOutMax=[]  PParamMin=[]  PParamMax=[]  IParamMin=[]  IParamMax=[]  DParamMin=[]  DParamMax=[]  NParamMin=[]  NParamMax=[]  KbParamMin=[]  KbParamMax=[]  KtParamMin=[]  KtParamMax=[]  KbOutMin=[]  KbOutMax=[]  KtOutMin=[]  KtOutMax=[]  IntegratorOutMin=[]  IntegratorOutMax=[]  FilterOutMin=[]  FilterOutMax=[]  SumI1OutMin=[]  SumI1OutMax=[]  SumI2OutMin=[]  SumI2OutMax=[]  SumI3OutMin=[]  SumI3OutMax=[]  SumI4OutMin=[]  SumI4OutMax=[]  SumDOutMin=[]  SumDOutMax=[]  DifferentiatorOutMin=[]  DifferentiatorOutMax=[]  FilterDiffOutCoefMin=[]  FilterDiffOutCoefMax=[]  ReciprocalOutMin=[]  ReciprocalOutMax=[]  SumDenOutMin=[]  SumDenOutMax=[]  SumNumOutMin=[]  SumNumOutMax=[]  DivideOutMin=[]  DivideOutMax=[]  UdiffTsProdOutMin=[]  UdiffTsProdOutMax=[]  NTsProdOutMin=[]  NTsProdOutMax=[]  UintegralTsProdOutMin=[]  UintegralTsProdOutMax=[]  UngainTsProdOutMin=[]  UngainTsProdOutMax=[]  IntegratorContinuousStateAttributes=''  IntegratorStateMustResolveToSignalObject=off  IntegratorRTWStateStorageClass=Auto  FilterContinuousStateAttributes=''  FilterStateMustResolveToSignalObject=off  FilterRTWStateStorageClass=Auto  ParallelPVariant=InternalParameters  IdealPVariant=Disabled  IVariant=InternalParameters  DVariant=InternalParameters  IntegratorVariant=Continuous  SatVariant=Enabled  AWVariant=ContClampingParallel  PCopyVariant=Disabled  TRVariant=Disabled  FdbkBlocksVariant=Forward  IdealPFdbkVariant=Disabled  SatFdbkVariant=Disabled  DerivativeFilterVariant=ContFilter  NVariant=InternalParameters  NCopyVariant=Disabled  FilterICVariant=InternalICsFilter  IntegratorICVariant=InternalICs  ExternalResetVariant=Disabled  TRSumVariant=Passthrough  SumFdbkVariant=Disabled  SumVariant=Sum_PID  TsampFilterVariant=InternalTs  TsampNgainVariant=Passthrough  TsampIntegralVariant=Passthrough  ExternalSaturationOutDataTypeStr=Inherit: Same as second input
  Product : Product
  Subtract : Sum  Inputs=+-
  Sum : Sum  Inputs=|++
  Terminator : Terminator
  Acc Reference : Outport
  wires:
  Ego Speed/1 -> Product/2
  Time Headway/1 -> Product/1
  Default Spacing/1 -> Sum/1
  Product/1 -> Sum/2
  Sum/1 -> Subtract/2
  Relative Distance/1 -> Subtract/1
  Subtract/1 -> PID Controller/1
  PID Controller/1 -> Acc Reference/1
  Relative Speed/1 -> Terminator/1
